simulink library "libGeodesy"  (R2022b)
settings: Solver=ode45  StartTime=0.0  StopTime=10.0  RelTol=1e-3  EnableMultiTasking=on
undefined symbols (not defined in the file): SimIn
libraries: libMathOperations x2, $bdroot x1
settings Model: Creator=eheim  LastModifiedBy=macheson
settings SolverCC: AlgebraicLoopSolver=TrustRegion
settings DataIOCC: LimitDataPoints=on  SaveFormat=Array  SignalLoggingSaveFormat=ModelDataLogs  ReturnWorkspaceOutputs=off
settings OptimizationCC: ExpressionDepthLimit=2147483647  LifeSpan=inf
settings DebuggingCC: UnderspecifiedInitializationDetection=Classic  MergeDetectMultiDrivingBlocksExec=none  SolverPrmCheckMsg=warning  FcnCallInpInsideContextMsg=warning  UnconnectedInputMsg=warning  UnconnectedOutputMsg=warning  UnconnectedLineMsg=warning  StateNameClashWarn=warning  SFUnexpectedBacktrackingDiag=warning  SFNoUnconditionalDefaultTransitionDiag=warning  SFExecutionAtInitializationDiag=none  SFMachineParentedDataDiag=warning  ArithmeticOperatorsInVariantConditions=warning
settings HardwareCC: ProdBitPerPointer=32  ProdBitPerSizeT=32  ProdBitPerPtrDiffT=32  ProdLargestAtomicFloat=None  ProdIntDivRoundTo=Undefined  ProdEndianess=Unspecified  ProdWordSize=32  ProdHWDeviceType=32-bit Generic
settings ModelReferenceCC: EnableRefExpFcnMdlSchedulingChecks=on  PropagateSignalLabelsOutOfModel=off
settings SFSimCC: SimUseLocalCustomCode=off  CustomCodeUndefinedFunction=UseInterfaceOnly
settings RTWCC: RTWUseLocalCustomCode=off  DLArmComputeVersion=19.05
settings CodeAppCC: StateflowObjectComments=on
settings GRTTargetCC: TargetLangStandard=C89/C90 (ANSI)  CombineOutputUpdateFcns=off  GRTInterface=on
settings ConfigComp: CovMetricSettings=dw  CovSaveCumulativeToWorkspaceVar=on  CovSaveSingleToWorkspaceVar=on  CovExternalEMLEnable=off  CovSFcnEnable=off

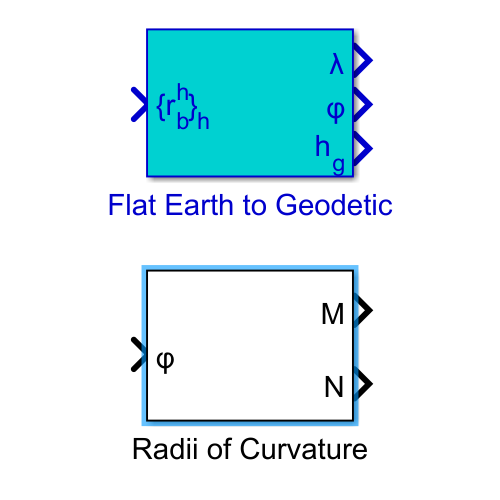
[thumbnail: Simulink's stored preview of the top-level diagram]
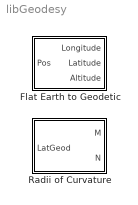
== system libGeodesy ==
  Flat Earth to Geodetic : Subsystem  mask(Flat Earth to Geodetic){lat=SimIn.IC.LatGeod, lon=SimIn.IC.Lon, a=SimIn.Environment.Earth.RadiusEquator, e=SimIn.Environment.Earth.Eccentricity}
      mask prompts: lat "Initial geodetic latitude (radians)"; lon "Initial longitude (radians)"; a "Planet semi-major axis radius"; e "Planet eccentricity"
      mask help: Estimates geodetic latitude, longitude and altitude from change in North-East-Down position. Input position units must match units of planet parmeters.
      mask Display:
      | port_label('input',1,'\{r_b^h\}_h','texmode','on')
      | port_label('output',1,'\lambda','texmode','on')
      | port_label('output',2,'\phi','texmode','on')
      | port_label('output',3,'h_g','texmode','on')
  Radii of Curvature : Subsystem  mask(Radii of Curvature){a=SimIn.Environment.Earth.RadiusEquator, e=SimIn.Environment.Earth.Eccentricity}
      mask prompts: a "Semi-major axis radius"; e "Eccentricity"
      mask help: Computes the radii of curvature for the ellipsoid
      mask Display:
      | port_label('input',1,'\phi','texmode','on')
      | port_label('output',1,'M','texmode','on')
      | port_label('output',2,'N','texmode','on')

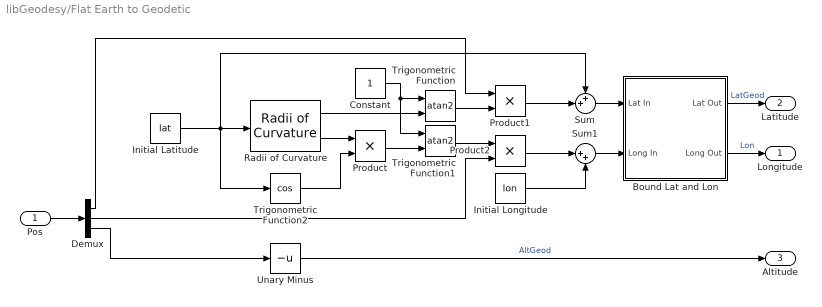
== system libGeodesy/Flat Earth to Geodetic ==
  Pos : Inport
  Bound Lat and Lon : Subsystem
  Constant : Constant
  Demux : Demux  Outputs=3
  Initial Latitude : Constant  Value=lat
  Initial Longitude : Constant  Value=lon
  Product : Product  RndMeth=Zero
  Product1 : Product  RndMeth=Zero
  Product2 : Product  RndMeth=Zero
  Radii of Curvature : $bdroot/Radii of Curvature  a=a  e=e
  Sum : Sum  Inputs=++|
  Sum1 : Sum  Inputs=|++
  Trigonometric Function : Trigonometry  Operator=atan2
  Trigonometric Function1 : Trigonometry  Operator=atan2
  Trigonometric Function2 : Trigonometry  Operator=cos
  Unary Minus : UnaryMinus
  Longitude : Outport
  Latitude : Outport  Port=2
  Altitude : Outport  Port=3
  wires:
  Radii of Curvature/2 -> Product/1
  Initial Latitude/1 -> Radii of Curvature/1, Trigonometric Function2/1, Sum/1
  Trigonometric Function2/1 -> Product/2
  Initial Longitude/1 -> Sum1/2
  Trigonometric Function/1 -> Product1/2
  Radii of Curvature/1 -> Trigonometric Function/2
  Constant/1 -> Trigonometric Function/1, Trigonometric Function1/1
  Product/1 -> Trigonometric Function1/2
  Trigonometric Function1/1 -> Product2/1
  Pos/1 -> Demux/1
  Demux/1 -> Product1/1
  Demux/2 -> Product2/2
  Demux/3 -> Unary Minus/1
  Unary Minus/1 -> Altitude/1  "AltGeod"
  Product1/1 -> Sum/2
  Product2/1 -> Sum1/1
  Sum/1 -> Bound Lat and Lon/1(Lat In)
  Sum1/1 -> Bound Lat and Lon/2(Long In)
  Bound Lat and Lon/1(Lat Out) -> Latitude/1  "LatGeod"
  Bound Lat and Lon/2(Long Out) -> Longitude/1  "Lon"

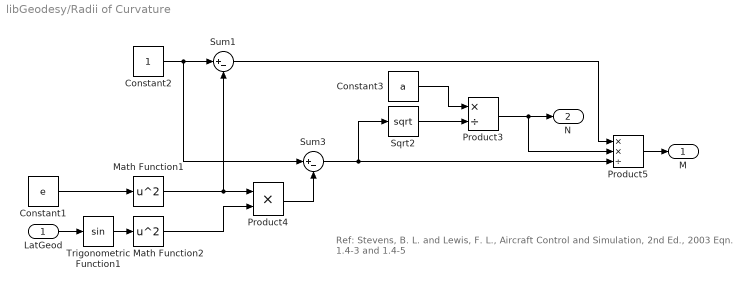
== system libGeodesy/Radii of Curvature ==
  note: Ref: Stevens, B. L. and Lewis, F. L., Aircraft Control and Simulation, 2nd Ed., 2003
      | Eqn. 1.4-3 and 1.4-5
  LatGeod : Inport
  Constant1 : Constant  Value=e
  Constant2 : Constant
  Constant3 : Constant  Value=a
  Math Function1 : Math  Operator=square  SignedPower=on
  Math Function2 : Math  Operator=square  SignedPower=on
  Product3 : Product  Inputs=*/  RndMeth=Zero
  Product4 : Product  RndMeth=Zero
  Product5 : Product  Inputs=**/  RndMeth=Zero
  Sqrt2 : Sqrt
  Sum1 : Sum  Inputs=|+-
  Sum3 : Sum  Inputs=|+-
  Trigonometric Function1 : Trigonometry
  M : Outport
  N : Outport  Port=2
  wires:
  LatGeod/1 -> Trigonometric Function1/1
  Constant1/1 -> Math Function1/1
  Product5/1 -> M/1
  Constant3/1 -> Product3/1
  Sum1/1 -> Product5/1
  Product3/1 -> N/1, Product5/2
  Sqrt2/1 -> Product3/2
  Sum3/1 -> Product5/3, Sqrt2/1
  Product4/1 -> Sum3/2
  Math Function2/1 -> Product4/2
  Trigonometric Function1/1 -> Math Function2/1
  Math Function1/1 -> Product4/1, Sum1/2
  Constant2/1 -> Sum3/1, Sum1/1

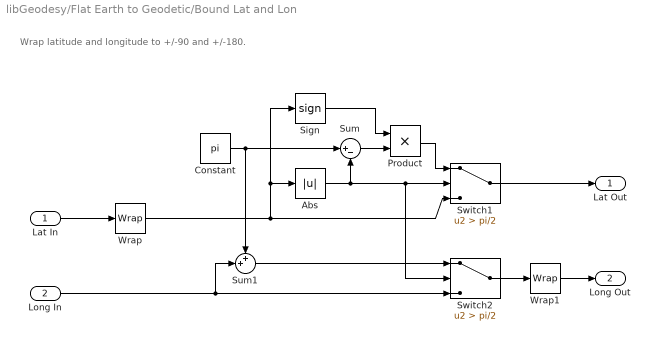
== system libGeodesy/Flat Earth to Geodetic/Bound Lat and Lon ==
  note: Wrap latitude and longitude to +/-90 and +/-180.
  Lat In : Inport
  Long In : Inport  Port=2
  Abs : Abs  SaturateOnIntegerOverflow=off
  Constant : Constant  Value=pi
  Product : Product  RndMeth=Zero
  Sign : Signum
  Sum : Sum  Inputs=|+-
  Sum1 : Sum  Inputs=++|
  Switch1 : Switch  Criteria=u2 > Threshold  Threshold=pi/2  SaturateOnIntegerOverflow=off  InputSameDT=off
  Switch2 : Switch  Criteria=u2 > Threshold  Threshold=pi/2  SaturateOnIntegerOverflow=off  InputSameDT=off
  Wrap : libMathOperations/Wrap  R=2*pi  M=-pi
  Wrap1 : libMathOperations/Wrap  R=2*pi  M=-pi
  Lat Out : Outport
  Long Out : Outport  Port=2
  wires:
  Wrap1/1 -> Long Out/1
  Abs/1 -> Switch2/2, Switch1/2, Sum/2
  Wrap/1 -> Switch1/3, Abs/1, Sign/1
  Long In/1 -> Switch2/3, Sum1/2
  Switch2/1 -> Wrap1/1
  Constant/1 -> Sum/1, Sum1/1
  Sum/1 -> Product/2
  Sign/1 -> Product/1
  Product/1 -> Switch1/1
  Sum1/1 -> Switch2/1
  Switch1/1 -> Lat Out/1
  Lat In/1 -> Wrap/1
